simulink model "uklad_michal"  (R2023a)
settings: Solver=FixedStepAuto  StartTime=0.0  StopTime=200  FixedStep=0.0001  MaxStep=0.001  MinStep=0.00001  RelTol=1e-3  EnableMultiTasking=on
undefined symbols (not defined in the file): A, A_act, B, B_act, C, C_act, D, D_act
libraries: slpidlib x2
settings Model: Creator=sinia  LastModifiedBy=Michal
settings SolverCC: InitialStep=0.00001  AllowMultiTaskInputOutput=on  ShapePreserveControl=EnableAll  PositivePriorityOrder=on

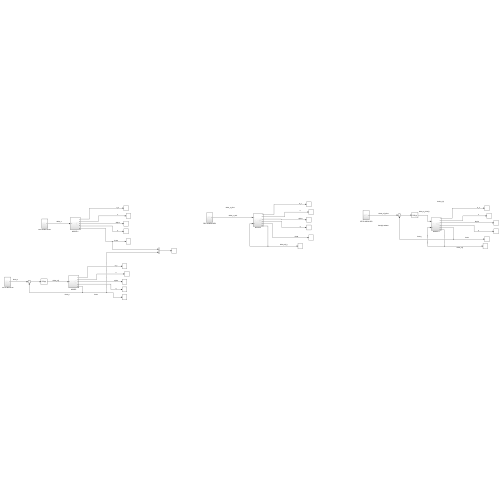
[thumbnail: Simulink's stored preview of the top-level diagram]
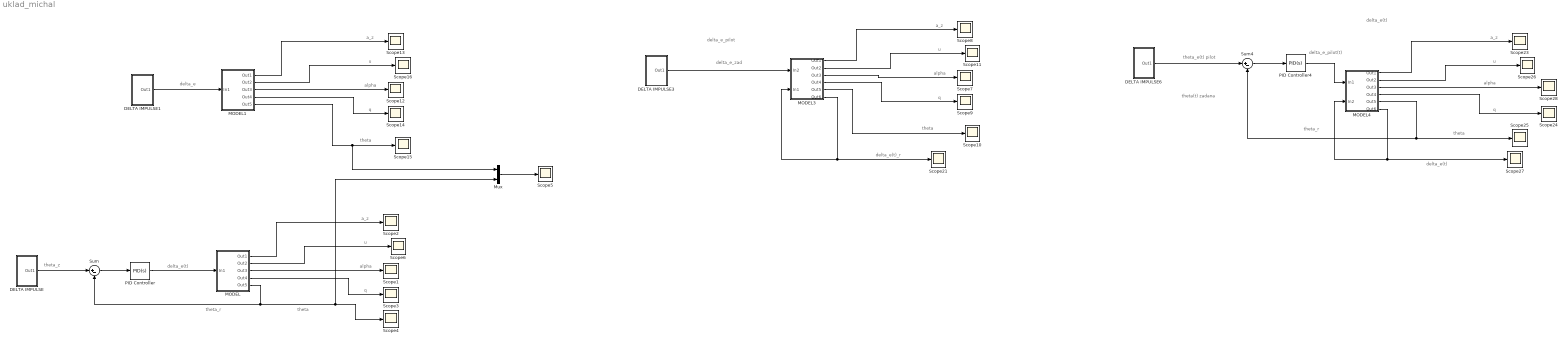
== system uklad_michal ==
  note: delta_e(t)
  note: theta_z
  note: theta
  note: u
  note: a_z
  note: q
  note: alpha
  note: theta_r
  note: theta
  note: alpha
  note: u
  note: delta_e
  note: a_z
  note: q
  note: a_z
  note: theta
  note: alpha
  note: q
  note: u
  note: delta_e_zad
  note: delta_e_pilot
  note: delta_e(t)_r
  note: delta_e_pilot(t)
  note: delta_e(t)
  note: a_z
  note: u
  note: theta(t) zadana
  note: theta_e(t) pilot
  note: q
  note: alpha
  note: theta
  note: delta_e(t)
  note: theta_r
  DELTA IMPULSE : Subsystem
  DELTA IMPULSE1 : Subsystem
  DELTA IMPULSE3 : Subsystem
  DELTA IMPULSE6 : Subsystem
  MODEL : Subsystem
  MODEL1 : Subsystem
  MODEL3 : Subsystem
  MODEL4 : Subsystem
  Mux : Mux  Inputs=2
  PID Controller : slpidlib/PID Controller  Controller=PID  Form=Parallel  TimeDomain=Continuous-time  UseExternalTs=off  SampleTime=-1  IntegratorMethod=Forward Euler  FilterMethod=Forward Euler  ControllerParametersSource=internal  P=-0.413800816220284  I=-0.000512729607222032  UseKiTs=off  D=2.94801931096674  N=0.140365707470412  UseFilter=on  TunerSelectOption=Transfer Function Based (PID Tuner App)  InitialConditionSource=internal  InitialConditionForIntegrator=0  InitialConditionForFilter=0  DifferentiatorICPrevScaledInput=0  ExternalReset=none  TrackingMode=off  Kt=1  LimitOutput=off  SatLimitsSource=internal  UpperSaturationLimit=inf  LowerSaturationLimit=-inf  LinearizeAsGain=on  AntiWindupMode=none  Kb=1  LimitIntegrator=off  UpperIntegratorSaturationLimit=inf  LowerIntegratorSaturationLimit=-inf  POutMin=[]  POutMax=[]  IOutMin=[]  IOutMax=[]  DOutMin=[]  DOutMax=[]  NOutMin=[]  NOutMax=[]  SumOutMin=[]  SumOutMax=[]  SaturationOutMin=[]  SaturationOutMax=[]  PParamMin=[]  PParamMax=[]  IParamMin=[]  IParamMax=[]  DParamMin=[]  DParamMax=[]  NParamMin=[]  NParamMax=[]  KbParamMin=[]  KbParamMax=[]  KtParamMin=[]  KtParamMax=[]  KbOutMin=[]  KbOutMax=[]  KtOutMin=[]  KtOutMax=[]  IntegratorOutMin=[]  IntegratorOutMax=[]  FilterOutMin=[]  FilterOutMax=[]  SumI1OutMin=[]  SumI1OutMax=[]  SumI2OutMin=[]  SumI2OutMax=[]  SumI3OutMin=[]  SumI3OutMax=[]  SumI4OutMin=[]  SumI4OutMax=[]  SumDOutMin=[]  SumDOutMax=[]  DifferentiatorOutMin=[]  DifferentiatorOutMax=[]  FilterDiffOutCoefMin=[]  FilterDiffOutCoefMax=[]  ReciprocalOutMin=[]  ReciprocalOutMax=[]  SumDenOutMin=[]  SumDenOutMax=[]  SumNumOutMin=[]  SumNumOutMax=[]  DivideOutMin=[]  DivideOutMax=[]  UdiffTsProdOutMin=[]  UdiffTsProdOutMax=[]  NTsProdOutMin=[]  NTsProdOutMax=[]  UintegralTsProdOutMin=[]  UintegralTsProdOutMax=[]  UngainTsProdOutMin=[]  UngainTsProdOutMax=[]  ClampingZeroOutDataTypeStr=Inherit: Inherit via back propagation  ClampingZeroOutMin=[]  ClampingZeroOutMax=[]  FilterDenConstantOutDataTypeStr=Inherit: Inherit via back propagation  FilterDenConstantOutMin=[]  FilterDenConstantOutMax=[]  PCopyOutDataTypeStr=Inherit: Inherit via back propagation  PCopyOutMin=[]  PCopyOutMax=[]  NCopyOutDataTypeStr=Inherit: Inherit via back propagation  NCopyOutMin=[]  NCopyOutMax=[]  IntegratorContinuousStateAttributes=''  IntegratorStateMustResolveToSignalObject=off  IntegratorRTWStateStorageClass=Auto  FilterContinuousStateAttributes=''  FilterStateMustResolveToSignalObject=off  FilterRTWStateStorageClass=Auto  ParallelPVariant=InternalParameters  IdealPVariant=Disabled  IVariant=InternalParameters  DVariant=InternalParameters  IntegratorVariant=Continuous  SatVariant=Disabled  AWVariant=Passthrough  PCopyVariant=Disabled  TRVariant=Disabled  FdbkBlocksVariant=Forward  IdealPFdbkVariant=Disabled  SatFdbkVariant=Disabled  DerivativeFilterVariant=ContFilter  NVariant=InternalParameters  NCopyVariant=Disabled  FilterICVariant=InternalICsFilter  IntegratorICVariant=InternalICs  ExternalResetVariant=Disabled  TRSumVariant=Passthrough  SumFdbkVariant=Disabled  SumVariant=Sum_PID  TsampFilterVariant=InternalTs  TsampNgainVariant=Passthrough  TsampIntegralVariant=Disabled_SignalSpec  ExternalSaturationOutDataTypeStr=Inherit: Same as second input
  PID Controller4 : slpidlib/PID Controller  Controller=PID  Form=Parallel  TimeDomain=Continuous-time  UseExternalTs=off  SampleTime=-1  IntegratorMethod=Forward Euler  FilterMethod=Forward Euler  ControllerParametersSource=internal  P=-0.413800816220284  I=-0.000512729607222032  UseKiTs=off  D=2.94801931096674  N=0.140365707470412  UseFilter=on  TunerSelectOption=Transfer Function Based (PID Tuner App)  InitialConditionSource=internal  InitialConditionForIntegrator=0  InitialConditionForFilter=0  DifferentiatorICPrevScaledInput=0  ExternalReset=none  TrackingMode=off  Kt=1  LimitOutput=off  SatLimitsSource=internal  UpperSaturationLimit=inf  LowerSaturationLimit=-inf  LinearizeAsGain=on  AntiWindupMode=none  Kb=1  LimitIntegrator=off  UpperIntegratorSaturationLimit=inf  LowerIntegratorSaturationLimit=-inf  POutMin=[]  POutMax=[]  IOutMin=[]  IOutMax=[]  DOutMin=[]  DOutMax=[]  NOutMin=[]  NOutMax=[]  SumOutMin=[]  SumOutMax=[]  SaturationOutMin=[]  SaturationOutMax=[]  PParamMin=[]  PParamMax=[]  IParamMin=[]  IParamMax=[]  DParamMin=[]  DParamMax=[]  NParamMin=[]  NParamMax=[]  KbParamMin=[]  KbParamMax=[]  KtParamMin=[]  KtParamMax=[]  KbOutMin=[]  KbOutMax=[]  KtOutMin=[]  KtOutMax=[]  IntegratorOutMin=[]  IntegratorOutMax=[]  FilterOutMin=[]  FilterOutMax=[]  SumI1OutMin=[]  SumI1OutMax=[]  SumI2OutMin=[]  SumI2OutMax=[]  SumI3OutMin=[]  SumI3OutMax=[]  SumI4OutMin=[]  SumI4OutMax=[]  SumDOutMin=[]  SumDOutMax=[]  DifferentiatorOutMin=[]  DifferentiatorOutMax=[]  FilterDiffOutCoefMin=[]  FilterDiffOutCoefMax=[]  ReciprocalOutMin=[]  ReciprocalOutMax=[]  SumDenOutMin=[]  SumDenOutMax=[]  SumNumOutMin=[]  SumNumOutMax=[]  DivideOutMin=[]  DivideOutMax=[]  UdiffTsProdOutMin=[]  UdiffTsProdOutMax=[]  NTsProdOutMin=[]  NTsProdOutMax=[]  UintegralTsProdOutMin=[]  UintegralTsProdOutMax=[]  UngainTsProdOutMin=[]  UngainTsProdOutMax=[]  ClampingZeroOutDataTypeStr=Inherit: Inherit via back propagation  ClampingZeroOutMin=[]  ClampingZeroOutMax=[]  FilterDenConstantOutDataTypeStr=Inherit: Inherit via back propagation  FilterDenConstantOutMin=[]  FilterDenConstantOutMax=[]  PCopyOutDataTypeStr=Inherit: Inherit via back propagation  PCopyOutMin=[]  PCopyOutMax=[]  NCopyOutDataTypeStr=Inherit: Inherit via back propagation  NCopyOutMin=[]  NCopyOutMax=[]  IntegratorContinuousStateAttributes=''  IntegratorStateMustResolveToSignalObject=off  IntegratorRTWStateStorageClass=Auto  FilterContinuousStateAttributes=''  FilterStateMustResolveToSignalObject=off  FilterRTWStateStorageClass=Auto  ParallelPVariant=InternalParameters  IdealPVariant=Disabled  IVariant=InternalParameters  DVariant=InternalParameters  IntegratorVariant=Continuous  SatVariant=Disabled  AWVariant=Passthrough  PCopyVariant=Disabled  TRVariant=Disabled  FdbkBlocksVariant=Forward  IdealPFdbkVariant=Disabled  SatFdbkVariant=Disabled  DerivativeFilterVariant=ContFilter  NVariant=InternalParameters  NCopyVariant=Disabled  FilterICVariant=InternalICsFilter  IntegratorICVariant=InternalICs  ExternalResetVariant=Disabled  TRSumVariant=Passthrough  SumFdbkVariant=Disabled  SumVariant=Sum_PID  TsampFilterVariant=InternalTs  TsampNgainVariant=Passthrough  TsampIntegralVariant=Disabled_SignalSpec  ExternalSaturationOutDataTypeStr=Inherit: Same as second input
  Scope{1..16,21,23..28} (23 alike) : Scope
  Sum : Sum  Inputs=|+-
  Sum4 : Sum  Inputs=|+-
  wires:
  DELTA IMPULSE/1(Out1) -> Sum/1
  PID Controller/1 -> MODEL/1(In1)
  MODEL/1(Out1) -> Scope2/1
  MODEL/2(Out2) -> Scope6/1
  MODEL/3(Out3) -> Scope1/1
  MODEL/4(Out4) -> Scope3/1
  Sum/1 -> PID Controller/1
  MODEL1/4(Out4) -> Scope14/1
  MODEL1/3(Out3) -> Scope12/1
  DELTA IMPULSE1/1(Out1) -> MODEL1/1(In1)
  MODEL1/1(Out1) -> Scope13/1
  MODEL1/2(Out2) -> Scope16/1
  MODEL3/1(Out1) -> Scope8/1
  MODEL3/2(Out2) -> Scope11/1
  MODEL3/5(Out5) -> Scope10/1
  MODEL3/4(Out4) -> Scope9/1
  MODEL3/3(Out3) -> Scope7/1
  MODEL3/6(Out6) -> Scope21/1, MODEL3/2(In1)
  MODEL4/4(Out4) -> Scope24/1
  MODEL4/1(Out1) -> Scope23/1
  MODEL4/5(Out5) -> Sum4/2, Scope25/1
  MODEL4/2(Out2) -> Scope26/1
  PID Controller4/1 -> MODEL4/1(In1)
  MODEL4/3(Out3) -> Scope28/1
  Sum4/1 -> PID Controller4/1
  DELTA IMPULSE6/1(Out1) -> Sum4/1
  MODEL4/6(Out6) -> MODEL4/2(In2), Scope27/1
  DELTA IMPULSE3/1(Out1) -> MODEL3/1(In2)
  MODEL/5(Out5) -> Mux/2, Scope4/1, Sum/2
  MODEL1/5(Out5) -> Mux/1, Scope15/1
  Mux/1 -> Scope5/1

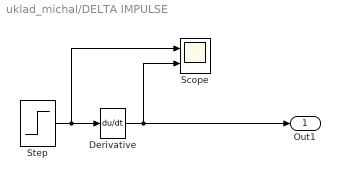
== system uklad_michal/DELTA IMPULSE ==
  Derivative : Derivative
  Scope : Scope  NumInputPorts=2
  Step : Step  SampleTime=0
  Out1 : Outport
  wires:
  Step/1 -> Scope/1, Derivative/1
  Derivative/1 -> Out1/1, Scope/2

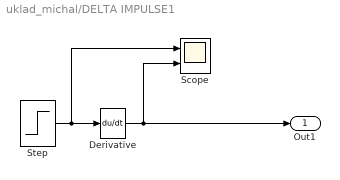
== system uklad_michal/DELTA IMPULSE1 ==
  Derivative : Derivative
  Scope : Scope  NumInputPorts=2
  Step : Step  SampleTime=0
  Out1 : Outport
  wires:
  Step/1 -> Scope/1, Derivative/1
  Derivative/1 -> Out1/1, Scope/2

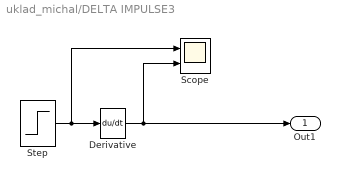
== system uklad_michal/DELTA IMPULSE3 ==
  Derivative : Derivative
  Scope : Scope  NumInputPorts=2
  Step : Step  SampleTime=0
  Out1 : Outport
  wires:
  Step/1 -> Scope/1, Derivative/1
  Derivative/1 -> Out1/1, Scope/2

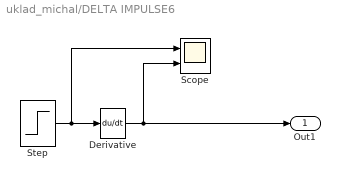
== system uklad_michal/DELTA IMPULSE6 ==
  Derivative : Derivative
  Scope : Scope  NumInputPorts=2
  Step : Step  SampleTime=0
  Out1 : Outport
  wires:
  Step/1 -> Scope/1, Derivative/1
  Derivative/1 -> Out1/1, Scope/2

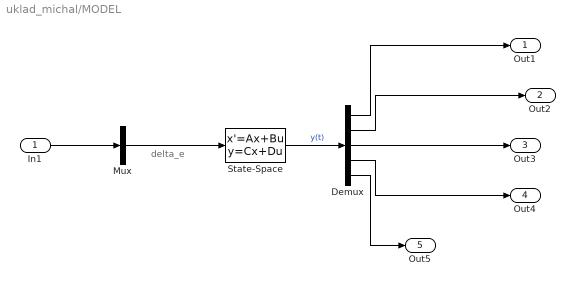
== system uklad_michal/MODEL ==
  note: delta_e
  In1 : Inport
  Demux : Demux  Outputs=5
  Mux : Mux  Inputs=1
  State-Space : StateSpace  A=A  B=B  C=C  D=D  InitialCondition=0
  Out1 : Outport
  Out2 : Outport  Port=2
  Out3 : Outport  Port=3
  Out4 : Outport  Port=4
  Out5 : Outport  Port=5
  wires:
  In1/1 -> Mux/1
  State-Space/1 -> Demux/1  "y(t)"
  Mux/1 -> State-Space/1
  Demux/5 -> Out5/1
  Demux/2 -> Out2/1
  Demux/1 -> Out1/1
  Demux/3 -> Out3/1
  Demux/4 -> Out4/1

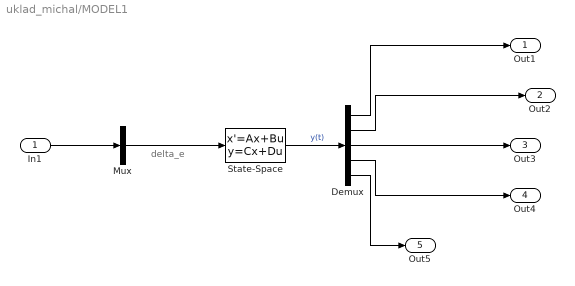
== system uklad_michal/MODEL1 ==
  note: delta_e
  In1 : Inport
  Demux : Demux  Outputs=5
  Mux : Mux  Inputs=1
  State-Space : StateSpace  A=A  B=B  C=C  D=D  InitialCondition=0
  Out1 : Outport
  Out2 : Outport  Port=2
  Out3 : Outport  Port=3
  Out4 : Outport  Port=4
  Out5 : Outport  Port=5
  wires:
  In1/1 -> Mux/1
  State-Space/1 -> Demux/1  "y(t)"
  Mux/1 -> State-Space/1
  Demux/5 -> Out5/1
  Demux/2 -> Out2/1
  Demux/1 -> Out1/1
  Demux/3 -> Out3/1
  Demux/4 -> Out4/1

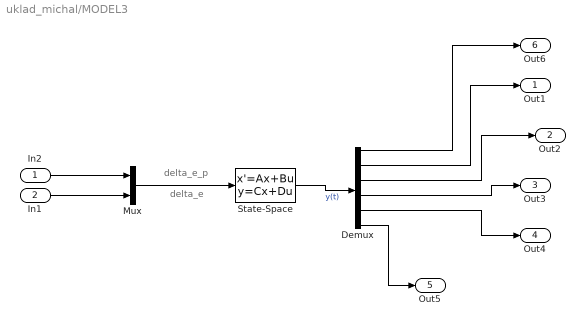
== system uklad_michal/MODEL3 ==
  note: delta_e
  note: delta_e_p
  In2 : Inport
  In1 : Inport  Port=2
  Demux : Demux  Outputs=6
  Mux : Mux  Inputs=2
  State-Space : StateSpace  A=A_act  B=B_act  C=C_act  D=D_act  InitialCondition=0
  Out1 : Outport
  Out2 : Outport  Port=2
  Out3 : Outport  Port=3
  Out4 : Outport  Port=4
  Out5 : Outport  Port=5
  Out6 : Outport  Port=6
  wires:
  In1/1 -> Mux/2
  State-Space/1 -> Demux/1  "y(t)"
  Mux/1 -> State-Space/1
  Demux/6 -> Out5/1
  Demux/3 -> Out2/1
  Demux/2 -> Out1/1
  Demux/4 -> Out3/1
  Demux/5 -> Out4/1
  In2/1 -> Mux/1
  Demux/1 -> Out6/1

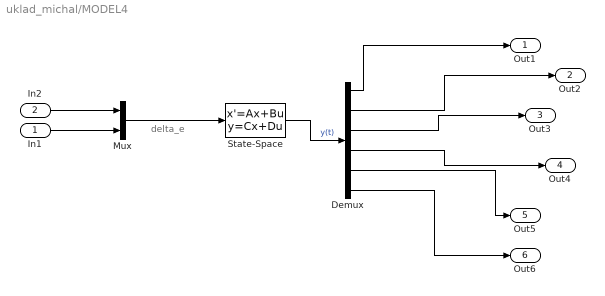
== system uklad_michal/MODEL4 ==
  note: delta_e
  In1 : Inport
  In2 : Inport  Port=2
  Demux : Demux  Outputs=6
  Mux : Mux  Inputs=2
  State-Space : StateSpace  A=A_act  B=B_act  C=C_act  D=D_act  InitialCondition=0
  Out1 : Outport
  Out2 : Outport  Port=2
  Out3 : Outport  Port=3
  Out4 : Outport  Port=4
  Out5 : Outport  Port=5
  Out6 : Outport  Port=6
  wires:
  In1/1 -> Mux/2
  State-Space/1 -> Demux/1  "y(t)"
  Mux/1 -> State-Space/1
  Demux/5 -> Out5/1
  Demux/2 -> Out2/1
  Demux/1 -> Out1/1
  Demux/3 -> Out3/1
  Demux/4 -> Out4/1
  Demux/6 -> Out6/1
  In2/1 -> Mux/1
